simulink model "TST_InterpolationAndLookup"  (Simulink 10.0)
settings: Solver=FixedStepDiscrete  StartTime=0.0  StopTime=10.0  FixedStep=.1  RelTol=1e-3  EnableMultiTasking=on
undefined symbols (not defined in the file): TST_LookupData_BreakPointsX1D, TST_LookupData_BreakPointsX2D, TST_LookupData_BreakPointsY2D, TST_LookupData_DataPoints1D, TST_LookupData_DataPoints2D
settings Model: Creator=mcasey  LastModifiedBy=unknown
settings DataIOCC: ExternalInput=[t,u]  LimitDataPoints=on  SignalLoggingSaveFormat=ModelDataLogs
settings OptimizationCC: BlockReduction=off  ConditionallyExecuteInputs=off  ExpressionDepthLimit=2147483647
settings DebuggingCC: SolverPrmCheckMsg=warning  FcnCallInpInsideContextMsg=warning  StateNameClashWarn=warning
settings GRTTargetCC: GeneratePreprocessorConditionals=Disable all
settings ConfigComp: CovExternalEMLEnable=off

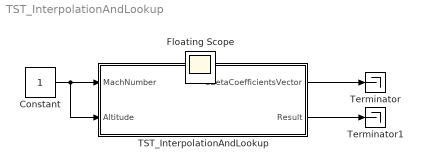
== system TST_InterpolationAndLookup ==
  Constant : Constant
  TST_InterpolationAndLookup : Subsystem  TreatAsAtomicUnit=on
  Terminator : Terminator
  Terminator1 : Terminator
  Floating Scope : Scope
  wires:
  Constant/1 -> TST_InterpolationAndLookup/1(MachNumber), TST_InterpolationAndLookup/2(Altitude)
  TST_InterpolationAndLookup/1(CBetaCoefficientsVector) -> Terminator/1
  TST_InterpolationAndLookup/2(Result) -> Terminator1/1

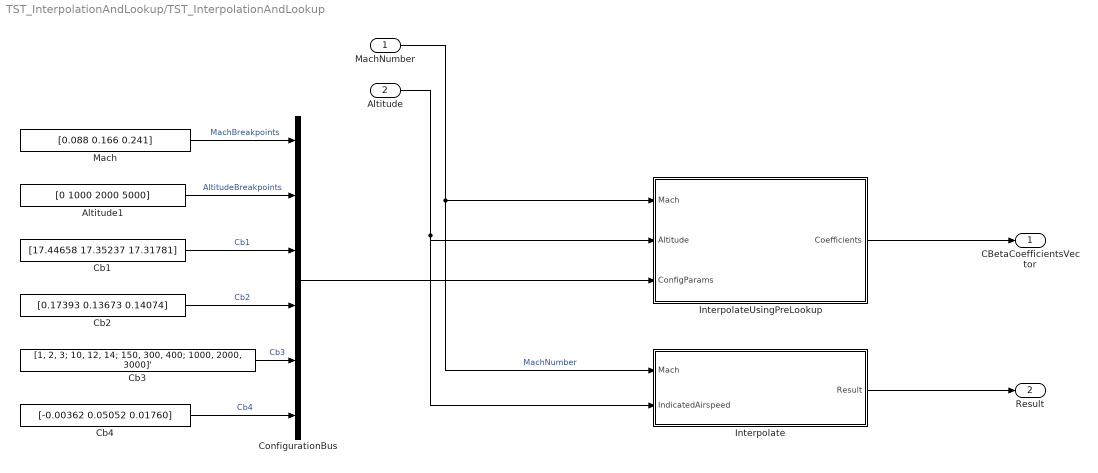
== system TST_InterpolationAndLookup/TST_InterpolationAndLookup ==
  MachNumber : Inport  OutDataTypeStr=double  PortDimensions=1
  Altitude : Inport  Port=2  OutDataTypeStr=double  PortDimensions=1
  Altitude1 : Constant  Value=[0 1000 2000 5000]
  Cb1 : Constant  Value=[17.44658 17.35237 17.31781]
  Cb2 : Constant  Value=[0.17393 0.13673 0.14074]
  Cb3 : Constant  Value=[1, 2, 3; 10, 12, 14; 150, 300, 400; 1000, 2000, 3000]'
  Cb4 : Constant  Value=[-0.00362 0.05052 0.01760]
  ConfigurationBus : BusCreator  Inputs=6
  Interpolate : Subsystem  TreatAsAtomicUnit=on
  InterpolateUsingPreLookup : Subsystem  TreatAsAtomicUnit=on
  Mach : Constant  Value=[0.088 0.166 0.241]
  CBetaCoefficientsVector : Outport  OutDataTypeStr=double  PortDimensions=4
  Result : Outport  Port=2  OutDataTypeStr=double  PortDimensions=1
  wires:
  Mach/1 -> ConfigurationBus/1  "MachBreakpoints"
  Altitude1/1 -> ConfigurationBus/2  "AltitudeBreakpoints"
  Cb1/1 -> ConfigurationBus/3  "Cb1"
  Cb2/1 -> ConfigurationBus/4  "Cb2"
  Cb3/1 -> ConfigurationBus/5  "Cb3"
  Cb4/1 -> ConfigurationBus/6  "Cb4"
  MachNumber/1 -> InterpolateUsingPreLookup/1(Mach), Interpolate/1(Mach)  "MachNumber"
  ConfigurationBus/1 -> InterpolateUsingPreLookup/3(ConfigParams)
  InterpolateUsingPreLookup/1(Coefficients) -> CBetaCoefficientsVector/1
  Altitude/1 -> InterpolateUsingPreLookup/2(Altitude), Interpolate/2(IndicatedAirspeed)
  Interpolate/1(Result) -> Result/1

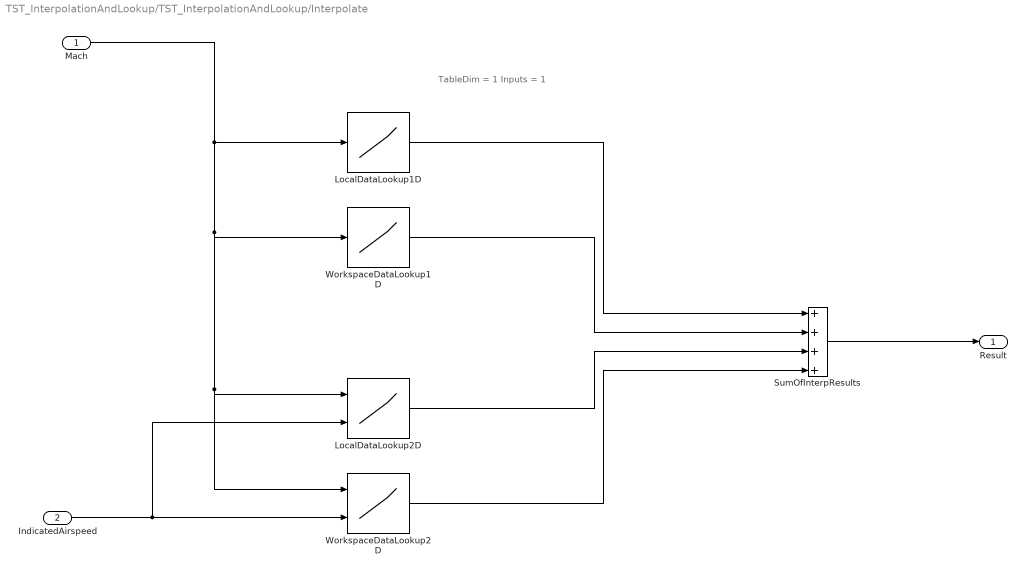
== system TST_InterpolationAndLookup/TST_InterpolationAndLookup/Interpolate ==
  note: TableDim = 1
      | Inputs = 1
  Mach : Inport
  IndicatedAirspeed : Inport  Port=2  OutDataTypeStr=double  PortDimensions=1
  LocalDataLookup1D : Lookup_n-D  NumberOfTableDimensions=1  BreakpointsForDimension1=[10 20 30]  Table=[1 2 3]  RndMeth=Simplest  InputSameDT=on
  LocalDataLookup2D : Lookup_n-D  BreakpointsForDimension1=[1 2 3 4]  BreakpointsForDimension2=[10 20 30]  Table=[1, 2, 3; 10, 20, 30; 25, 26, 27; 100, 200, 300]  RndMeth=Simplest  InputSameDT=on
  SumOfInterpResults : Sum  Inputs=++++
  WorkspaceDataLookup1D : Lookup_n-D  NumberOfTableDimensions=1  BreakpointsForDimension1=TST_LookupData_BreakPointsX1D  Table=TST_LookupData_DataPoints1D  RndMeth=Simplest  InputSameDT=on
  WorkspaceDataLookup2D : Lookup_n-D  BreakpointsForDimension1=TST_LookupData_BreakPointsY2D  BreakpointsForDimension2=TST_LookupData_BreakPointsX2D  Table=TST_LookupData_DataPoints2D  RndMeth=Simplest  InputSameDT=on
  Result : Outport
  wires:
  IndicatedAirspeed/1 -> WorkspaceDataLookup2D/2, LocalDataLookup2D/2
  Mach/1 -> LocalDataLookup1D/1, WorkspaceDataLookup1D/1, LocalDataLookup2D/1, WorkspaceDataLookup2D/1
  LocalDataLookup1D/1 -> SumOfInterpResults/1
  WorkspaceDataLookup1D/1 -> SumOfInterpResults/2
  WorkspaceDataLookup2D/1 -> SumOfInterpResults/4
  LocalDataLookup2D/1 -> SumOfInterpResults/3
  SumOfInterpResults/1 -> Result/1

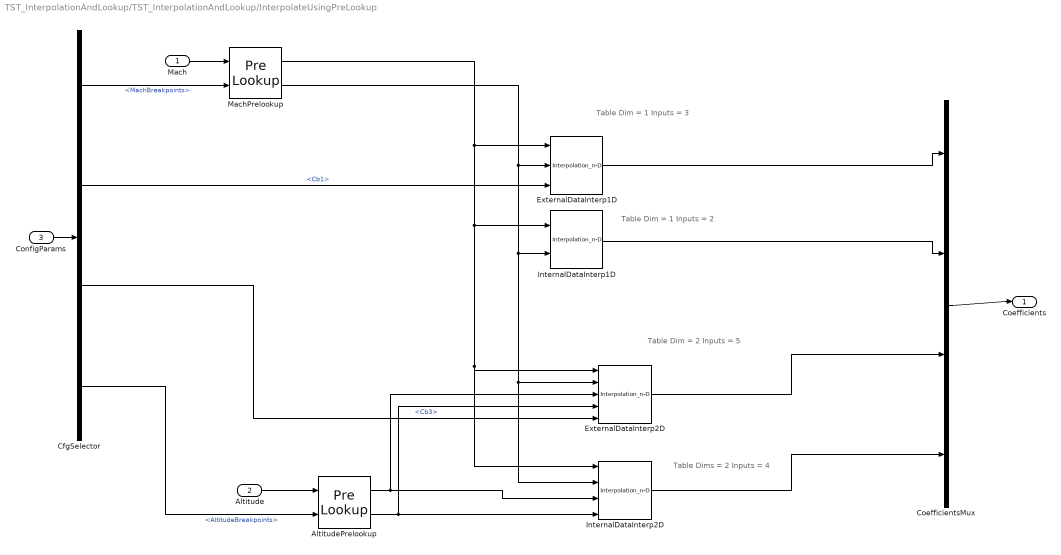
== system TST_InterpolationAndLookup/TST_InterpolationAndLookup/InterpolateUsingPreLookup ==
  note: Table Dim = 1
      | Inputs = 3
  note: Table Dim = 2
      | Inputs = 5
  note: Table Dim = 1
      | Inputs = 2
  note: Table Dims = 2
      | Inputs = 4
  Mach : Inport
  Altitude : Inport  Port=2  OutDataTypeStr=double  PortDimensions=1
  ConfigParams : Inport  Port=3
  AltitudePrelookup : PreLookup  BreakpointsDataSource=Input port  BreakpointsData=[10:10:110]  ExtrapMethod=Linear
      settings: InputPortMap=u0,p1
  CfgSelector : BusSelector  OutputSignals=MachBreakpoints,Cb1,Cb3,AltitudeBreakpoints
  CoefficientsMux : Mux
  ExternalDataInterp1D : Interpolation_n-D  NumberOfTableDimensions=1  TableSource=Input port  ExtrapMethod=Clip
      settings: InputPortMap=u0,u1,p2
  ExternalDataInterp2D : Interpolation_n-D  TableSource=Input port  ExtrapMethod=Clip
      settings: InputPortMap=u0,u1,u2,u3,p2
  InternalDataInterp1D : Interpolation_n-D  NumberOfTableDimensions=1  Table=[0.17393 0.13673 0.14074]  ExtrapMethod=Clip
      settings: InputPortMap=u0,u1
  InternalDataInterp2D : Interpolation_n-D  Table=[1, 2, 3; 10, 12, 14; 150, 300, 400; 1000, 2000, 3000]'  ExtrapMethod=Clip
  MachPrelookup : PreLookup  BreakpointsDataSource=Input port  BreakpointsData=[10:10:110]  ExtrapMethod=Linear
      settings: InputPortMap=u0,p1
  Coefficients : Outport
  wires:
  CfgSelector/1 -> MachPrelookup/2  "<MachBreakpoints>"
  InternalDataInterp1D/1 -> CoefficientsMux/2
  ExternalDataInterp1D/1 -> CoefficientsMux/1
  Mach/1 -> MachPrelookup/1
  ConfigParams/1 -> CfgSelector/1
  CoefficientsMux/1 -> Coefficients/1
  MachPrelookup/1 -> ExternalDataInterp1D/1, InternalDataInterp1D/1, InternalDataInterp2D/1, ExternalDataInterp2D/1
  MachPrelookup/2 -> ExternalDataInterp1D/2, InternalDataInterp1D/2, ExternalDataInterp2D/2, InternalDataInterp2D/2
  Altitude/1 -> AltitudePrelookup/1
  CfgSelector/2 -> ExternalDataInterp1D/3  "<Cb1>"
  CfgSelector/3 -> ExternalDataInterp2D/5  "<Cb3>"
  ExternalDataInterp2D/1 -> CoefficientsMux/3
  InternalDataInterp2D/1 -> CoefficientsMux/4
  CfgSelector/4 -> AltitudePrelookup/2  "<AltitudeBreakpoints>"
  AltitudePrelookup/2 -> InternalDataInterp2D/4, ExternalDataInterp2D/4
  AltitudePrelookup/1 -> InternalDataInterp2D/3, ExternalDataInterp2D/3
